simulink library "dspsolvers"  (Simulink 6.0)
libraries: dspsolvers x6, dspmtrx3 x4, dspfactors x3, dspinverses x1
settings Model: CovMetricSettings=d  Creator=dlinebar  LastModifiedBy=mlongfri  ExtModeAutoUpdateStatusClock=off  ProdHWDeviceType=Specified

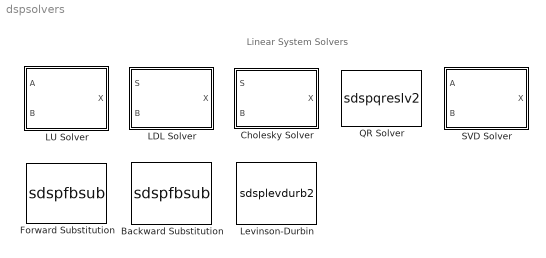
== system dspsolvers ==
  note: Linear System Solvers
  Backward Substitution : S-Function  FunctionName=sdspfbsub  Parameters=unit,1  mask(Backward Substitution){unit=off}
      mask prompts: unit "Force input to be unit-upper triangular"
      mask help: Solve UX=B where U is an upper (or unit-upper) triangular matrix. U must be square. B must have the same number of rows as U.
      mask init:
      | x=[ 0.45 0.45 0.18 0.45 NaN 0.495 0.585 0.585 0.495 0.495 NaN 0.63 0.675 NaN 0.63 0.675 NaN 0.72 0.81 0.81 0.72 0.72 ];
      | y=[ 0.1 0.7 0.7 0.1 NaN 0.1 0.1 0.7 0.7 0.1 NaN 0.35 0.35 NaN 0.45 0.45 NaN 0.1 0.1 0.7 0.7 0.1 ];
      mask Help: web(dspbhelp);
      mask Display:
      | plot(x,y); text(.4,0.9,'U X = B');
      | port_label('input',1,'U');
      | port_label('input',2,'B');
      | port_label('output',1,'X');
  Cholesky Solver : Subsystem  mask(Cholesky Solver){errmode=Warning}
      mask prompts: errmode "Non-positive definite input:"
      mask help: Solve SX=B using Cholesky factorization. S must be a square, symmetric (Hermitian) positive definite matrix. B must have the same number of rows as S.
      mask init:
      | x=[ 0.135 0.475 .475 0.135 0.135 NaN .135 .475 NaN 0.55 0.64 0.64 0.55  0.55 NaN 0.685 0.73 NaN 0.685 0.73 NaN 0.775 0.865 0.865 0.775 0.775 ];
      | y=[ 0.2 0.2 0.7 0.7 .2 NaN .7 .2 NaN 0.2 0.2 0.7 0.7 0.2 NaN 0.4 0.4 NaN 0.45 0.45 NaN 0.2 0.2 0.7 0.7 0.2 ];
      | set_param([gcb '/Cholesky Factorization'],'MaskTunableValues', {'off'});
      | set_param([gcb '/Cholesky Factorization'],'errmode',get_param(gcb,'errmode'));
      mask Help: web(dspbhelp);
      mask StyleString: popup(Ignore|Warning|Error)
      mask Display:
      | plot(x,y+0.05);
      | text(0.17,0.9,'SX=B (Chol)');
      | text(0.12,0.15,'[m x m]');
  Forward Substitution : S-Function  FunctionName=sdspfbsub  Parameters=unit,0  mask(Forward Substitution){unit=off}
      mask prompts: unit "Force input to be unit-lower triangular"
      mask help: Solve LX=B where L is a lower (or unit-lower) triangular matrix. L must be square. B must have the same number of rows as L.
      mask init:
      | x=[ 0.18 0.45 0.18 0.18 NaN 0.495 0.585 0.585 0.495 0.495 NaN 0.63 0.675 NaN 0.63 0.675 NaN 0.72 0.81 0.81 0.72 0.72 ];
      | y=[ 0.1 0.1 0.7 0.1 NaN 0.1 0.1 0.7 0.7 0.1 NaN 0.35 0.35 NaN 0.45 0.45 NaN 0.1 0.1 0.7 0.7 0.1 ];
      mask Help: web(dspbhelp);
      mask Display:
      | plot(x,y); text(.4,0.9,'L X = B');
      | port_label('input',1,'L');
      | port_label('input',2,'B');
      | port_label('output',1,'X');
  LDL Solver : Subsystem  mask(LDL Solver){errmode=Warning}
      mask prompts: errmode "Non-positive definite input:"
      mask help: Solve SX=B using LDL' factorization. Only for use with a symmetric (Hermitian) positive definite input matrix S. S must be square. B must have the same number of rows as S.
      mask init:
      | Bcols=1;
      | x=[ 0.135 0.475 .475 0.135 0.135 NaN .135 .475 NaN 0.55 0.64 0.64 0.55 0.55 NaN 0.685 0.73 NaN 0.685 0.73 NaN 0.775 0.865 0.865 0.775 0.775 ];
      | y=[ 0.2 0.2 0.7 0.7 0.2 NaN .7 .2 NaN 0.2 0.2 0.7 0.7 0.2 NaN 0.4 0.4 NaN 0.45 0.45 NaN 0.2 0.2 0.7 0.7 0.2 ];
      | set_param([gcb '/LDL Factorization'],'MaskTunableValues', {'off'});
      | set_param([gcb '/LDL Factorization'],'errmode',get_param(gcb,'errmode'));
      mask Help: web(dspbhelp);
      mask StyleString: popup(Ignore|Warning|Error)
      mask Display:
      | plot(x,y+0.05);
      | text(0.17,0.9,'SX=B (LDL'')');
      | text(0.12,0.15,'[m x m]');
  LU Solver : Subsystem  mask(LU Solver){}
      mask help: Solve AX=B using LU decomposition. A must be square. B must have the same number of rows as A.
      mask init:
      | x=[ 0.135 .475 0.475 0.135 .135 NaN 0.55 0.64 0.64 0.55 0.55 NaN 0.685 0.73 NaN 0.685 0.73 NaN 0.775 0.865 0.865 0.775 0.775 ];
      | y=[ 0.2 0.2 0.7 0.7 0.2 NaN 0.2 0.2 0.7 0.7 0.2 NaN 0.4 0.4 NaN 0.45 0.45 NaN 0.2 0.2 0.7 0.7 0.2 ];
      mask Help: web(dspbhelp);
      mask Display:
      | plot(x,y+0.05);
      | 
      | text(0.25,0.9,'AX=B (LU)');
      | 
      | text(0.12,0.15,'[m x m]');
  Levinson-Durbin : S-Function  DialogController=dspDDGCreate  DialogControllerArgs=DataTag0  FunctionName=sdsplevdurb2  Parameters=coeffOutFcn,outP,zeroInpHandling,dtInfo.firstCoeffMode,dtInfo.firstCoeffWordLength,dtInfo.firstCoeffFracLength,dtInfo.secondCoeffMode,dtInfo.secondCoeffWordLength,dtInfo.secondCoeffFracLength,dtInfo.prodOutputMode,dtInfo.prodOutputWordLength,dtInfo.prodOutputFracLength,dtInfo.accumMode,dtInfo.accumWordLength,dtInfo.accumFracLength,dtInfo.outputMode,dtInfo.outputWordLength,dtInfo.outputFracLength,dtInfo.roundingMode,dtInfo.overflowMode  mask(Levinson-Durbin){coeffOutFcn=K, outP=off, zeroInpHandling=on, additionalParams=off, allowOverrides=off, firstCoeffMode=Binary point scaling, firstCoeffWordLength=16, firstCoeffFracLength=15, secondCoeffMode=Binary point scaling, secondCoeffWordLength=16, secondCoeffFracLength=15, outputMode=Same as input, outputWordLength=16, outputFracLength=15, accumMode=Same as input, accumWordLength=32, accumFracLength=30, prodOutputMode=Same as input, prodOutputWordLength=32, prodOutputFracLength=30, roundingMode=Floor, overflowMode=off}
      mask prompts: coeffOutFcn "Output(s):"; outP "Output prediction error power (P)"; zeroInpHandling "If the value of lag 0 is zero, A=[1 zeros], K=[zeros], P=0"; additionalParams "--------------- Show additional parameters ---------------"; allowOverrides "Allow overrides from DSP Attributes blocksAllow overrides from DSP Attributes blocks"; firstCoeffMode "Fixed-point A attributes:"; firstCoeffWordLength "A word length:"; firstCoeffFracLength "A fraction length:"; secondCoeffMode "Fixed-point K attributes:"; secondCoeffWordLength "K word length:"; secondCoeffFracLength "K fraction length:"; outputMode "Fixed-point P attributes:"; outputWordLength "P word length:"; outputFracLength "P fractional length:"; accumMode "Fixed-point accumulator attributes:"; accumWordLength "Accumulator word length:"; accumFracLength "Accumulator fraction length:"; prodOutputMode "Fixed-point product output attributes:"; prodOutputWordLength "Product output word length:"; prodOutputFracLength "Product output fraction length:"; roundingMode "Round integer calculations towards:"; overflowMode "Saturate on integer overflow"
      mask help: Solve Hermitian Toeplitz system of equations using the Levinson-Durbin recursion. Input is typically a vector of autocorrelation coefficients with lag 0 as the first element. Outputs polynomial coefficients A, reflection coefficients K, and/or the prediction error power P.
      mask init:
      | s = dspblklevdurb2('setup', coeffOutFcn, outP);
      | 
      | dtInfo = dspblklevdurb2('init');
      settings: CopyFcn=dspfixptcopycallback
      mask Help: web(dspbhelp);
      mask StyleString: popup(A and K|A|K),checkbox,checkbox,checkbox,checkbox,popup(Binary point scaling|Slope and bias scaling|User-defined),edit,edit,popup(Binary point scaling|Slope and bias scaling|User-defined),edit,edit,popup(Same as input|Binary point scaling|Slope and bias scaling|User-defined),edit,edit,popup(Same as product output|Same as input|Binary point scaling|Slope and bias scaling|User-defined),edit,edit,popup(Same as input|Binary point scaling|Slope and bias scaling|User-defined),edit,edit,popup(Floor|Nearest),checkbox
      mask Display:
      | text(0.2,0.6,'Levinson-');
      | text(0.3,0.4,'Durbin');
      | port_label('output',s.o1,s.o1s);
      | port_label('output',s.o2,s.o2s);
      | port_label('output',s.o3,s.o3s);
  QR Solver : S-Function  FunctionName=sdspqreslv2  mask(QR Solver){}
      mask help: Solve AX=B using QR factorization. B must have the same number of rows as A. If A is not square, the output is a least squares solution.
      mask init:
      | x=[ 0.2 0.475 .475 0.2 0.2 NaN 0.55 0.64 0.64 0.55 0.55 NaN 0.685 0.73 NaN 0.685 0.73 NaN 0.775 0.865 0.865 0.775 0.775 ];
      | y=[ 0.2 0.2 0.7 0.7 0.2 NaN 0.35 0.35 0.7 0.7 0.35 NaN 0.4 0.4 NaN 0.45 0.45 NaN 0.2 0.2 0.7 0.7 0.2 ];
      mask Help: web(dspbhelp);
      mask Display:
      | plot(x,y+0.05);
      | text(0.23,0.9,'AX=B (QR)');
      | text(0.17,0.15,'[m x n]');
      | port_label('input',1,'A');
      | port_label('input',2,'B');
      | port_label('output',1,'X');
  SVD Solver : Subsystem  mask(SVD Solver){}
      mask help: Solve AX=B using Singular Value Decomposition. B must have the same number of rows as A. If A is not square, the output is a least squares solution.
      mask init: same as dspsolvers/QR Solver
      mask Help: web(dspbhelp);
      mask Display:
      | plot(x,y+0.05);
      | 
      | text(0.2,0.9,'AX=B (SVD)');
      | 
      | text(0.17,0.15,'[m x n]');

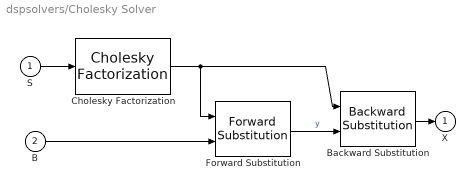
== system dspsolvers/Cholesky Solver ==
  S : Inport
  B : Inport  Port=2
  Backward Substitution : dspsolvers/Backward Substitution  unit=off
  Cholesky Factorization : dspfactors/Cholesky Factorization  errmode=Warning
  Forward Substitution : dspsolvers/Forward Substitution  unit=off
  X : Outport  InitialOutput=0
  wires:
  S/1 -> Cholesky Factorization/1
  Forward Substitution/1 -> Backward Substitution/2  "y"
  Backward Substitution/1 -> X/1
  B/1 -> Forward Substitution/2
  Cholesky Factorization/1 -> Forward Substitution/1, Backward Substitution/1

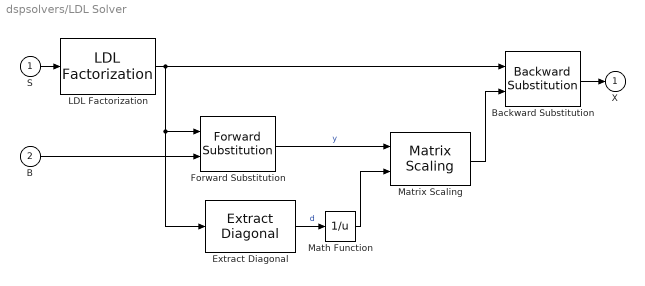
== system dspsolvers/LDL Solver ==
  S : Inport
  B : Inport  Port=2
  Backward Substitution : dspsolvers/Backward Substitution  unit=on
  Extract Diagonal : dspmtrx3/Extract Diagonal
  Forward Substitution : dspsolvers/Forward Substitution  unit=on
  LDL Factorization : dspfactors/LDL Factorization  errmode=Warning
  Math Function : Math  Operator=reciprocal  SaturateOnIntegerOverflow=on
  Matrix Scaling : dspmtrx3/Matrix Scaling  mode=Scale rows (D*A)  D_Source=Input port  D_VectFromMask=[0.5 0.25]  roundingMode=Floor  overflowMode=off
  X : Outport  InitialOutput=0
  wires:
  Backward Substitution/1 -> X/1
  LDL Factorization/1 -> Backward Substitution/1, Forward Substitution/1, Extract Diagonal/1
  B/1 -> Forward Substitution/2
  S/1 -> LDL Factorization/1
  Forward Substitution/1 -> Matrix Scaling/1  "y"
  Matrix Scaling/1 -> Backward Substitution/2
  Extract Diagonal/1 -> Math Function/1  "d"
  Math Function/1 -> Matrix Scaling/2

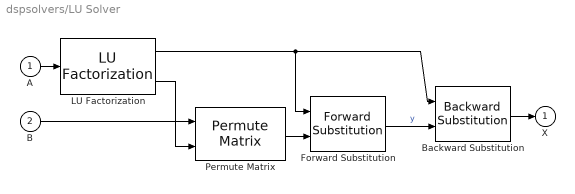
== system dspsolvers/LU Solver ==
  A : Inport
  B : Inport  Port=2
  Backward Substitution : dspsolvers/Backward Substitution  unit=off
  Forward Substitution : dspsolvers/Forward Substitution  unit=on
  LU Factorization : dspfactors/LU Factorization  singular=off
  Permute Matrix : dspmtrx3/Permute Matrix  mode=Rows  ZeroOneIdxMode=One-based  errmode=Clip Index  checkDims=on
  X : Outport  InitialOutput=0
  wires:
  A/1 -> LU Factorization/1
  Permute Matrix/1 -> Forward Substitution/2
  Backward Substitution/1 -> X/1
  Forward Substitution/1 -> Backward Substitution/2  "y"
  B/1 -> Permute Matrix/1
  LU Factorization/2 -> Permute Matrix/2
  LU Factorization/1 -> Forward Substitution/1, Backward Substitution/1

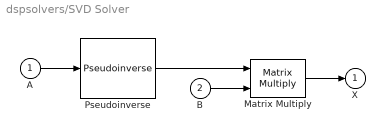
== system dspsolvers/SVD Solver ==
  A : Inport
  B : Inport  Port=2
  Matrix Multiply : dspmtrx3/Matrix Multiply  numInputPorts=2  OptimizationLevel=None
  Pseudoinverse : dspinverses/Pseudoinverse
  X : Outport  InitialOutput=0
  wires:
  A/1 -> Pseudoinverse/1
  Pseudoinverse/1 -> Matrix Multiply/1
  Matrix Multiply/1 -> X/1
  B/1 -> Matrix Multiply/2
